simulink model "StepDownChopperWithFilterRLoad"  (R2015b)
settings: Solver=FixedStepAuto  StartTime=0.0  StopTime=.1  FixedStep=1/(X*fs)  RelTol=1e-3
values from neighbouring files (symbols this model uses):
  Cf = 10e-6    (= 1e-05)    [StepDownChopperWithFilterRLoadCode.m]
  D = 0.4    [StepDownChopperWithFilterRLoadCode.m]
  fs = 30000    [StepDownChopperWithFilterRLoadCode.m]
  Lf = 5e-4    (= 0.0005)    [StepDownChopperWithFilterRLoadCode.m]
  R = 4.8    [StepDownChopperWithFilterRLoadCode.m]
  Vd = 32    [StepDownChopperWithFilterRLoadCode.m]
  X = 100    [StepDownChopperWithFilterRLoadCode.m]
libraries: powerlib x11
settings Model: Creator=Akshay Laturkar  LastModifiedBy=Sourabh Suri

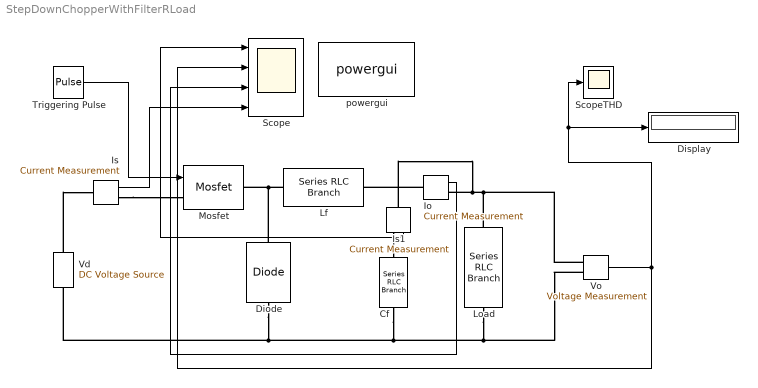
== system StepDownChopperWithFilterRLoad ==
  Cf : powerlib/Elements/Series RLC Branch  LConnTagsString=__new0  RConnTagsString=__new0  BranchType=C  Resistance=1  Inductance=Lf  SetiL0=off  InitialCurrent=0  Capacitance=Cf  Setx0=off  InitialVoltage=0  Measurements=None
  Diode : powerlib/Power Electronics/Diode  Ron=0.001  Lon=0  Vf=0.8  IC=0  UseSnubber=off  Rs=500  Cs=250e-9  Measurements=off
  Display : Display
  Io : powerlib/Measurements/Current Measurement  PhasorSimulation=off  OutputType=Complex  PSBequivalent=0
  Is : powerlib/Measurements/Current Measurement  PhasorSimulation=off  OutputType=Complex  PSBequivalent=0
  Is1 : powerlib/Measurements/Current Measurement  PhasorSimulation=off  OutputType=Complex  PSBequivalent=0
  Lf : powerlib/Elements/Series RLC Branch  LConnTagsString=__new0  RConnTagsString=__new0  BranchType=RL  Resistance=0.07  Inductance=Lf  SetiL0=off  InitialCurrent=0  Capacitance=1e-6  Setx0=off  InitialVoltage=0  Measurements=None
  Load : powerlib/Elements/Series RLC Branch  LConnTagsString=__new0  RConnTagsString=__new0  BranchType=R  Resistance=R  Inductance=1e-3  SetiL0=off  InitialCurrent=0  Capacitance=1e-6  Setx0=off  InitialVoltage=0  Measurements=None
  Mosfet : powerlib/Power Electronics/Mosfet  Ron=0.1  Lon=0  Rd=0.01  Vfd=0  IC=0  Rs=1e5  Cs=inf  Measurements=off
  Scope : Scope  NumInputPorts=4
  ScopeTHD : Scope
  Triggering Pulse : DiscretePulseGenerator  PulseType=Time based  Period=1/fs  PulseWidth=D*100
  Vd : powerlib/Electrical Sources/DC Voltage Source  Amplitude=Vd  Measurements=None
  Vo : powerlib/Measurements/Voltage Measurement  PhasorSimulation=off  OutputType=Complex  PSBequivalent=0
  powergui : powerlib/powergui  Priority=1  SimulationMode=Discrete  SolverType=Tustin/Backward Euler (TBE)  SampleTime=1/(X*fs)  frequency=60  SPID=off  DisableSnubberDevices=off  DisableRonSwitches=off  DisableVfSwitches=off  SwTol=0  DisplayEquations=off  Interpol=off  ExternalGateDelay=off  methode=off  Ts=10  FunctionMessages=off  echomessages=off  HookPort=off  EnableUseOfTLC=off  x0status=blocks  frequencyindice=0  Pbase=100e6  ErrMax=1e-4  Iterations=50  UnitsV=kV  UnitsW=MW  buscounter=0  RestoreLinks=warning  ResistiveCurrentMeasurement=off  Frange=[0:2:500]  Ylog=off  Xlog=on  ShowGrid=off  save=off  variable=ZData  structure=Vo  ZoomFFT=off  StartTime=0.6  cycles=1000  DisplayStyle=5  fundamental=100000  FreqAxis=off  MaxFrequency=1000000  frequencyindicesteady=1  RmsSteady=1  display=off
  wires:
  Triggering Pulse/1 -> Mosfet/1
  Vo/1 -> Display/1, ScopeTHD/1, Scope/2
  Io/1 -> Scope/3
  Is/1 -> Scope/4
  Is1/1 -> Scope/1
  connections:
  Vo/LConn2 -- Load/RConn1 -- Cf/RConn1 -- Diode/LConn1 -- Vd/LConn1
  Lf/LConn1 -- Diode/RConn1 -- Mosfet/RConn1
  Is/RConn1 -- Mosfet/LConn1
  Vd/RConn1 -- Is/LConn1
  Load/LConn1 -- Vo/LConn1 -- Is1/LConn1 -- Io/RConn1
  Is1/RConn1 -- Cf/LConn1
  Io/LConn1 -- Lf/RConn1
